simulink model "Practica_3"  (R2024b)
settings: Solver=VariableStepAuto  StartTime=0.0  StopTime=10.0  RelTol=1e-3
values from neighbouring files (symbols this model uses):
  b1 = 1000    [Practica.m]    (also in Practica_3.m)
  k1 = 16182    [Practica.m]    (also in Practica_3.m)
  k2 = 19000    [Practica.m]    (also in Practica_3.m)
  m1 = 290    [Practica.m]    (also in Practica_3.m)
  m2 = 59    [Practica.m]    (also in Practica_3.m)
settings Model: Creator=escor  LastModifiedBy=mac09
settings OptimizationCC: ReuseModelBlockBuffer=off
settings RTWCC: GPUComputeCapability=3.5

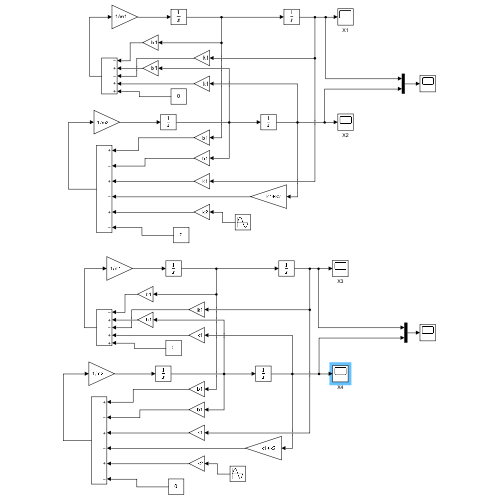
[thumbnail: Simulink's stored preview of the top-level diagram]
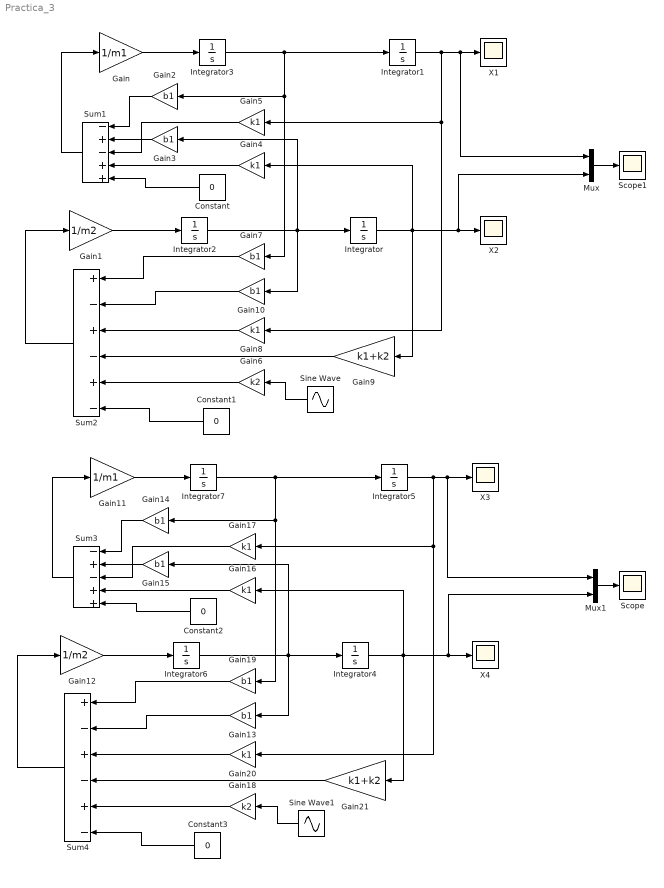
== system Practica_3 ==
  Constant{,1..3} (4 alike) : Constant  Value=0
  Gain : Gain  Gain=1/m1
  Gain1 : Gain  Gain=1/m2
  Gain{2..3,7,10,13..15,19} (8 alike) : Gain  Gain=b1
  Gain11 : Gain  Gain=1/m1
  Gain12 : Gain  Gain=1/m2
  Gain{4..5,8,16..17,20} (6 alike) : Gain  Gain=k1
  Gain18 : Gain  Gain=k2
  Gain21 : Gain  Gain=k1+k2
  Gain6 : Gain  Gain=k2
  Gain9 : Gain  Gain=k1+k2
  Integrator{,1..7} (8 alike) : Integrator
  Mux : Mux  Inputs=2
  Mux1 : Mux  Inputs=2
  Scope : Scope
  Scope1 : Scope
  Sine Wave : Sin  Amplitude=0.05  Frequency=0.5*pi  SampleTime=0
  Sine Wave1 : Sin  Amplitude=0.05  Frequency=20*pi  SampleTime=0
  Sum1 : Sum  Inputs=-+-++
  Sum2 : Sum  Inputs=+-+-+-
  Sum3 : Sum  Inputs=-+-++
  Sum4 : Sum  Inputs=+-+-+-
  X{1..4} (4 alike) : Scope
  wires:
  Sum2/1 -> Gain1/1
  Gain7/1 -> Sum2/1
  Sum1/1 -> Gain/1
  Integrator3/1 -> Gain7/1, Gain2/1, Integrator1/1
  Gain5/1 -> Sum1/3
  Gain9/1 -> Sum2/4
  Constant1/1 -> Sum2/6
  Gain4/1 -> Sum1/4
  Gain6/1 -> Sum2/5
  Sine Wave/1 -> Gain6/1
  Integrator2/1 -> Integrator/1, Gain10/1, Gain3/1
  Constant/1 -> Sum1/5
  Gain10/1 -> Sum2/2
  Integrator/1 -> Gain9/1, Mux/2, X2/1, Gain4/1
  Gain/1 -> Integrator3/1
  Gain8/1 -> Sum2/3
  Gain1/1 -> Integrator2/1
  Gain2/1 -> Sum1/1
  Gain3/1 -> Sum1/2
  Integrator1/1 -> Mux/1, X1/1, Gain8/1, Gain5/1
  Gain12/1 -> Integrator6/1
  Constant3/1 -> Sum4/6
  Gain15/1 -> Sum3/2
  Constant2/1 -> Sum3/5
  Integrator6/1 -> Integrator4/1, Gain13/1, Gain15/1
  Gain18/1 -> Sum4/5
  Sum3/1 -> Gain11/1
  Gain16/1 -> Sum3/4
  Integrator5/1 -> Mux1/1, X3/1, Gain20/1, Gain17/1
  Gain20/1 -> Sum4/3
  Gain14/1 -> Sum3/1
  Gain13/1 -> Sum4/2
  Gain11/1 -> Integrator7/1
  Gain19/1 -> Sum4/1
  Sum4/1 -> Gain12/1
  Gain17/1 -> Sum3/3
  Integrator7/1 -> Gain19/1, Gain14/1, Integrator5/1
  Gain21/1 -> Sum4/4
  Sine Wave1/1 -> Gain18/1
  Integrator4/1 -> Gain21/1, Mux1/2, X4/1, Gain16/1
  Mux1/1 -> Scope/1
  Mux/1 -> Scope1/1
